simulink model "ModeS_testbench_org"  (Simulink 10.0)
settings: Solver=VariableStepDiscrete  StartTime=0.0  StopTime=1e6  RelTol=1e-3
PreLoadFcn:
  | load data_Yb;
  | 
  | DataIn = Yb_with_time(:,2);
  | 
  | wl=16;
undefined symbols (not defined in the file): dfilt
libraries: simulink x27, dspobslib x2, dspsnks4 x2, hdlsllib x1, dspindex x1, dspsrcs4 x1
settings Model: Creator=mdonovan  LastModifiedBy=annonymous
settings DataIOCC: LimitDataPoints=on  SignalLoggingSaveFormat=ModelDataLogs  SaveOutput=off  SignalLogging=off  SaveTime=off
settings OptimizationCC: BlockReduction=off  BooleanDataType=off  ConditionallyExecuteInputs=off  DefaultParameterBehavior=Inlined  ExpressionDepthLimit=2147483647  LocalBlockOutputs=off
settings DebuggingCC: AlgebraicLoopMsg=error  SolverPrmCheckMsg=warning  SingleTaskRateTransMsg=error  FcnCallInpInsideContextMsg=warning  AllowSymbolicDim=off  StateNameClashWarn=warning
settings HardwareCC: ProdHWDeviceType=ASIC/FPGA->ASIC/FPGA  TargetBitPerLong=64  TargetBitPerPointer=64  TargetBitPerSizeT=64  TargetBitPerPtrDiffT=64  TargetLongLongMode=on  TargetIntDivRoundTo=Zero  TargetEndianess=LittleEndian  TargetWordSize=64  TargetHWDeviceType=MATLAB Host  ProdEqTarget=off
settings GRTTargetCC: GeneratePreprocessorConditionals=Disable all
settings ConfigComp: CovExternalEMLEnable=off

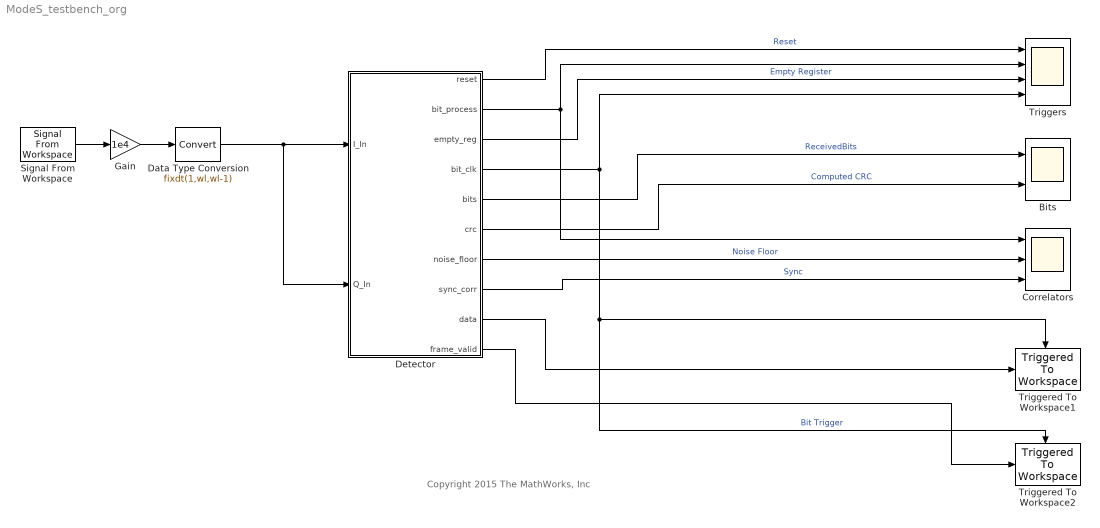
== system ModeS_testbench_org ==
  note: Copyright 2015 The MathWorks, Inc
  Bits : Scope  NumInputPorts=2
  Correlators : Scope  NumInputPorts=3
  Data Type Conversion : DataTypeConversion  OutDataTypeStr=fixdt(1,wl,wl-1)  LockScale=on
  Detector : Subsystem  TreatAsAtomicUnit=on
  Gain : Gain  Gain=1e4
  Signal From Workspace : dspsrcs4/Signal From Workspace  X=DataIn  Ts=1  nsamps=1  OutputAfterFinalValue=Setting to zero  ignoreOrWarnInputAndFrameLengths=off  OutputFrames=on
  Triggered To Workspace1 : dspsnks4/Triggered To Workspace  TriggerType=Rising edge  VariableName=data_out  Buffer=1000  Save2DMode=2-D array (concatenate along first dimension)
      settings: SourceProductName=DSP System Toolbox  SourceProductBaseCode=DS  FixptAsFi=off
  Triggered To Workspace2 : dspsnks4/Triggered To Workspace  TriggerType=Rising edge  VariableName=frame_valid  Buffer=1000  Save2DMode=2-D array (concatenate along first dimension)
      settings: SourceProductName=DSP System Toolbox  SourceProductBaseCode=DS  FixptAsFi=off
  Triggers : Scope  NumInputPorts=4
  wires:
  Signal From Workspace/1 -> Gain/1
  Data Type Conversion/1 -> Detector/1(I_In), Detector/2(Q_In)
  Gain/1 -> Data Type Conversion/1
  Detector/5(bits) -> Bits/1  "ReceivedBits"
  Detector/4(bit_clk) -> Triggered To Workspace2/Trigger, Triggered To Workspace1/Trigger, Triggers/4  "Bit Trigger"
  Detector/10(frame_valid) -> Triggered To Workspace2/1
  Detector/9(data) -> Triggered To Workspace1/1
  Detector/7(noise_floor) -> Correlators/2  "Noise Floor"
  Detector/6(crc) -> Bits/2  "Computed CRC"
  Detector/1(reset) -> Triggers/1  "Reset"
  Detector/2(bit_process) -> Triggers/2, Correlators/1
  Detector/3(empty_reg) -> Triggers/3  "Empty Register"
  Detector/8(sync_corr) -> Correlators/3  "Sync"

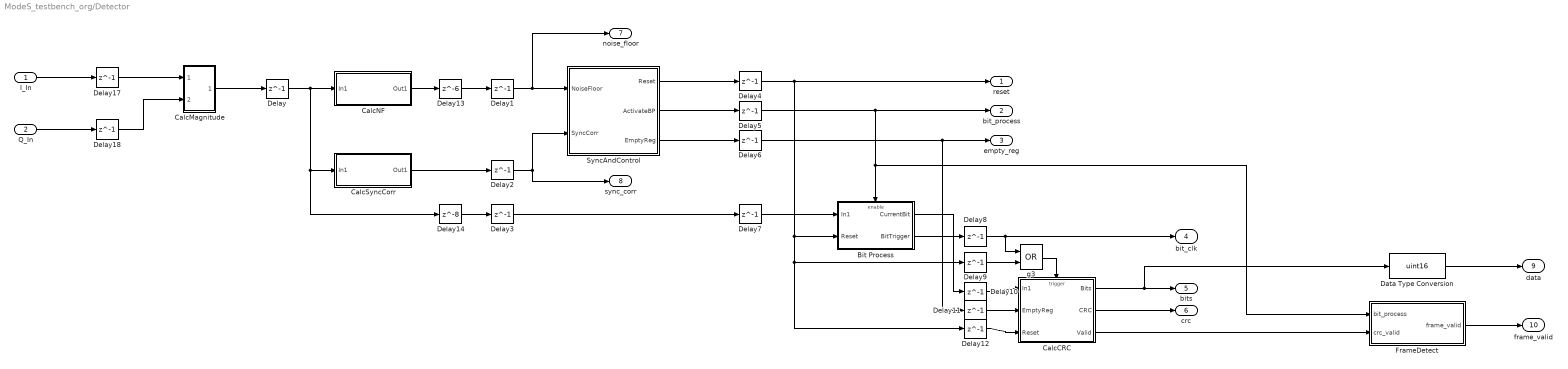
== system ModeS_testbench_org/Detector ==
  I_In : Inport
  Q_In : Inport  Port=2
  Bit Process : Subsystem  TreatAsAtomicUnit=on
  CalcCRC : Subsystem
  CalcMagnitude : Subsystem
  CalcNF : Subsystem
  CalcSyncCorr : Subsystem
  Data Type Conversion : DataTypeConversion  OutDataTypeStr=uint16
  Delay{,1..12,17..18} (15 alike) : Delay  DelayLength=1  InitialCondition=0  InputProcessing=Columns as channels (frame based)
  Delay13 : Delay  DelayLength=6  InitialCondition=0  InputProcessing=Columns as channels (frame based)
  Delay14 : Delay  DelayLength=8  InitialCondition=0  InputProcessing=Columns as channels (frame based)
  FrameDetect : Subsystem
  SyncAndControl : Stateflow chart  TreatAsAtomicUnit=on
  g3 : Logic  Operator=OR  AllPortsSameDT=off  OutDataTypeStr=boolean
  reset : Outport  VectorParamsAs1DForOutWhenUnconnected=off
  bit_process : Outport  Port=2  VectorParamsAs1DForOutWhenUnconnected=off
  empty_reg : Outport  Port=3  VectorParamsAs1DForOutWhenUnconnected=off
  bit_clk : Outport  Port=4  VectorParamsAs1DForOutWhenUnconnected=off
  bits : Outport  Port=5  VectorParamsAs1DForOutWhenUnconnected=off
  crc : Outport  Port=6  VectorParamsAs1DForOutWhenUnconnected=off
  noise_floor : Outport  Port=7  VectorParamsAs1DForOutWhenUnconnected=off
  sync_corr : Outport  Port=8  VectorParamsAs1DForOutWhenUnconnected=off
  data : Outport  Port=9  VectorParamsAs1DForOutWhenUnconnected=off
  frame_valid : Outport  Port=10  VectorParamsAs1DForOutWhenUnconnected=off
  wires:
  SyncAndControl/1(Reset) -> Delay4/1
  Bit Process/1(CurrentBit) -> Delay10/1
  SyncAndControl/3(EmptyReg) -> Delay6/1
  SyncAndControl/2(ActivateBP) -> Delay5/1
  Bit Process/2(BitTrigger) -> Delay8/1
  g3/1 -> CalcCRC/Trigger
  CalcNF/1(Out1) -> Delay13/1
  CalcSyncCorr/1(Out1) -> Delay2/1
  CalcCRC/1(Bits) -> Data Type Conversion/1, bits/1
  CalcCRC/2(CRC) -> crc/1
  Delay1/1 -> SyncAndControl/1(NoiseFloor), noise_floor/1
  Delay2/1 -> SyncAndControl/2(SyncCorr), sync_corr/1
  Delay3/1 -> Delay7/1
  Delay4/1 -> reset/1, Delay9/1, Delay12/1, Bit Process/2(Reset)
  Delay5/1 -> FrameDetect/1(bit_process), Bit Process/Enable, bit_process/1
  Delay6/1 -> empty_reg/1, Delay11/1
  Delay7/1 -> Bit Process/1(In1)
  Delay10/1 -> CalcCRC/1(In1)
  Delay11/1 -> CalcCRC/2(EmptyReg)
  Delay13/1 -> Delay1/1
  I_In/1 -> Delay17/1
  Q_In/1 -> Delay18/1
  Delay17/1 -> CalcMagnitude/1(In1)
  Delay18/1 -> CalcMagnitude/2(In2)
  CalcMagnitude/1(Out1) -> Delay/1
  Delay8/1 -> g3/1, bit_clk/1
  Delay12/1 -> CalcCRC/3(Reset)
  Delay9/1 -> g3/2
  CalcCRC/3(Valid) -> FrameDetect/2(crc_valid)
  FrameDetect/1(frame_valid) -> frame_valid/1
  Data Type Conversion/1 -> data/1
  Delay/1 -> CalcNF/1(In1), Delay14/1, CalcSyncCorr/1(In1)
  Delay14/1 -> Delay3/1

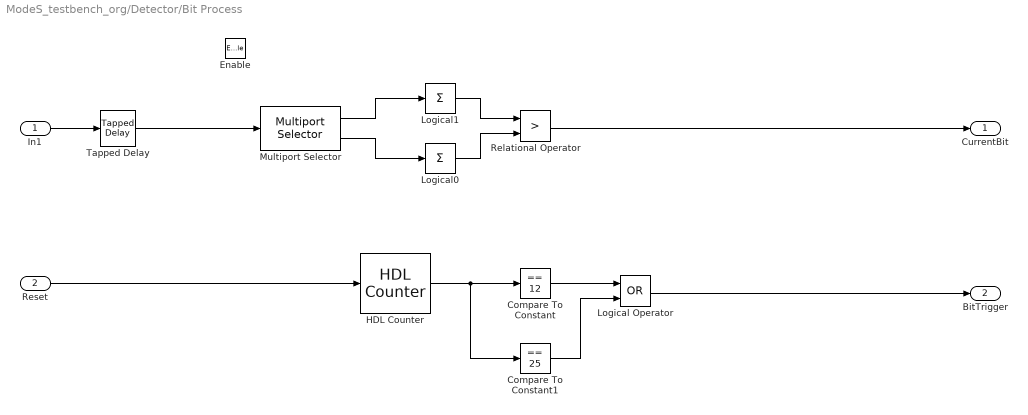
== system ModeS_testbench_org/Detector/Bit Process ==
  In1 : Inport
  Reset : Inport  Port=2
  Enable : EnablePort
  Compare To Constant : simulink/Logic and Bit Operations/Compare To Constant  relop===  const=12  OutDataTypeStr=boolean
  Compare To Constant1 : simulink/Logic and Bit Operations/Compare To Constant  relop===  const=25  OutDataTypeStr=boolean
  HDL Counter : hdlsllib/HDL Operations/HDL Counter  CountType=Count limited  CountInit=1  CountStep=1  CountMax=25  CountFromType=Initial value  CountFrom=1  CountResetPort=on  CountLoadPort=off  CountEnbPort=off  CountDirPort=off  CountDataType=Unsigned  CountWordLen=8  CountFracLen=0  CountSampTime=1
      settings: SourceProductName=HDL Coder  SourceProductBaseCode=HD
  Logical Operator : Logic  Operator=OR  AllPortsSameDT=off  OutDataTypeStr=boolean
  Logical0 : Sum  Inputs=+  AccumDataTypeStr=fixdt(1,wl,wl-3)  OutDataTypeStr=Inherit: Same as accumulator
  Logical1 : Sum  Inputs=+  AccumDataTypeStr=fixdt(1,wl,wl-3)  OutDataTypeStr=Inherit: Same as accumulator
  Multiport Selector : dspindex/Multiport Selector  rowsOrCols=Rows  idxCellArray={ 1:6,7:12}  idxErrMode=Clip Index
  Relational Operator : RelationalOperator  Operator=>  OutDataTypeStr=boolean  RndMeth=Nearest
  Tapped Delay : simulink/Discrete/Tapped Delay  vinit=0.0  samptime=1  NumDelays=12  DelayOrder=Oldest  includeCurrent=on
  CurrentBit : Outport  InitialOutput=0  VectorParamsAs1DForOutWhenUnconnected=off
  BitTrigger : Outport  Port=2  InitialOutput=0  VectorParamsAs1DForOutWhenUnconnected=off
  wires:
  Tapped Delay/1 -> Multiport Selector/1
  Multiport Selector/1 -> Logical1/1
  Multiport Selector/2 -> Logical0/1
  Logical1/1 -> Relational Operator/1
  Logical0/1 -> Relational Operator/2
  In1/1 -> Tapped Delay/1
  Relational Operator/1 -> CurrentBit/1
  Reset/1 -> HDL Counter/1
  HDL Counter/1 -> Compare To Constant/1, Compare To Constant1/1
  Compare To Constant/1 -> Logical Operator/1
  Compare To Constant1/1 -> Logical Operator/2
  Logical Operator/1 -> BitTrigger/1

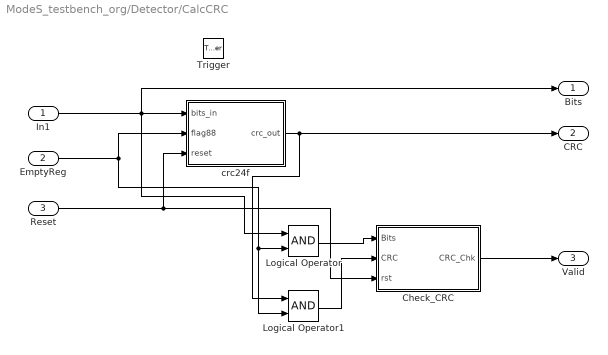
== system ModeS_testbench_org/Detector/CalcCRC ==
  In1 : Inport
  EmptyReg : Inport  Port=2
  Reset : Inport  Port=3
  Trigger : TriggerPort  VariantControl=Variant
  Check_CRC : Subsystem  TreatAsAtomicUnit=on
  Logical Operator : Logic  AllPortsSameDT=off  OutDataTypeStr=boolean
  Logical Operator1 : Logic  AllPortsSameDT=off  OutDataTypeStr=boolean
  crc24f : Subsystem
  Bits : Outport  InitialOutput=0  VectorParamsAs1DForOutWhenUnconnected=off
  CRC : Outport  Port=2  InitialOutput=0  VectorParamsAs1DForOutWhenUnconnected=off
  Valid : Outport  Port=3  InitialOutput=0  VectorParamsAs1DForOutWhenUnconnected=off
  wires:
  In1/1 -> Bits/1, Logical Operator/1, crc24f/1(bits_in)
  EmptyReg/1 -> crc24f/2(flag88), Logical Operator1/2, Logical Operator/2
  crc24f/1(crc_out) -> Logical Operator1/1, CRC/1
  Reset/1 -> Check_CRC/3(rst), crc24f/3(reset)
  Logical Operator/1 -> Check_CRC/1(Bits)
  Logical Operator1/1 -> Check_CRC/2(CRC)
  Check_CRC/1(CRC_Chk) -> Valid/1

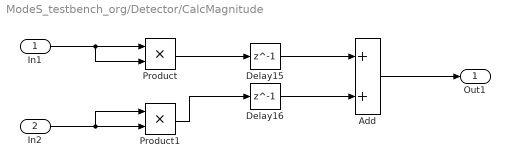
== system ModeS_testbench_org/Detector/CalcMagnitude ==
  In1 : Inport
  In2 : Inport  Port=2
  Add : Sum  OutDataTypeStr=fixdt(1,wl,wl-1)
  Delay15 : Delay  DelayLength=1  InitialCondition=0  InputProcessing=Columns as channels (frame based)
  Delay16 : Delay  DelayLength=1  InitialCondition=0  InputProcessing=Columns as channels (frame based)
  Product : Product  OutDataTypeStr=fixdt(1,wl,wl-1)
  Product1 : Product  OutDataTypeStr=fixdt(1,wl,wl-1)
  Out1 : Outport  VectorParamsAs1DForOutWhenUnconnected=off
  wires:
  Product/1 -> Delay15/1
  Product1/1 -> Delay16/1
  In1/1 -> Product/2, Product/1
  In2/1 -> Product1/1, Product1/2
  Delay15/1 -> Add/1
  Add/1 -> Out1/1
  Delay16/1 -> Add/2

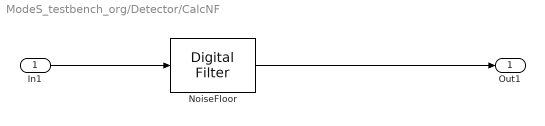
== system ModeS_testbench_org/Detector/CalcNF ==
  In1 : Inport
  NoiseFloor : dspobslib/Digital Filter  TypePopup=FIR (all zeros)  IIRFiltStruct=Direct form II transposed  AllPoleFiltStruct=Direct form  FIRFiltStruct=Direct form transposed  CoeffSource=Specify via dialog  NumCoeffs=(ones(64,1)/64)  DenCoeffs=[1 0.1]  BiQuadCoeffs=[1 0.3 0.4 1 0.1 0.2]  LatticeCoeffs=[0.2 0.4]  denIgnore=on  FiltPerSampPopup=One filter per frame  IC=0  ICnum=0  ICden=0  firstCoeffMode=Binary point scaling  firstCoeffWordLength=wl  firstCoeffFracLength=wl+4  outputMode=Binary point scaling  outputWordLength=wl  outputFracLength=wl  accumMode=Binary point scaling  accumWordLength=wl*2  accumFracLength=wl*2  prodOutputMode=Binary point scaling  prodOutputWordLength=wl*2  prodOutputFracLength=wl*2+5  roundingMode=Floor  overflowMode=off  ScaleValues=1  scaleValueFracLength=14  stageInFracLength=15  stageOutFracLength=15  FilterSource=Specify via dialog  dfiltObjectName=dfilt.dffir([1 2 1])  InputProcessing=Columns as channels (frame based)
      settings: SourceProductName=DSP System Toolbox  SourceProductBaseCode=DS
  Out1 : Outport  VectorParamsAs1DForOutWhenUnconnected=off
  wires:
  In1/1 -> NoiseFloor/1
  NoiseFloor/1 -> Out1/1

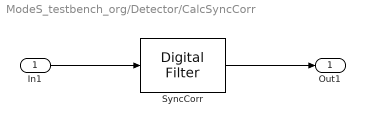
== system ModeS_testbench_org/Detector/CalcSyncCorr ==
  In1 : Inport
  SyncCorr : dspobslib/Digital Filter  TypePopup=FIR (all zeros)  IIRFiltStruct=Direct form II transposed  AllPoleFiltStruct=Direct form  FIRFiltStruct=Direct form  CoeffSource=Specify via dialog  NumCoeffs=|  DenCoeffs=[1 0.1]  BiQuadCoeffs=[1 0.3 0.4 1 0.1 0.2]  LatticeCoeffs=[0.2 0.4]  denIgnore=on  FiltPerSampPopup=One filter per frame  IC=0  ICnum=0  ICden=0  firstCoeffMode=Binary point scaling  firstCoeffWordLength=wl  firstCoeffFracLength=wl-2  outputMode=Binary point scaling  outputWordLength=wl  outputFracLength=wl-5  accumMode=Binary point scaling  accumWordLength=wl*2  accumFracLength=wl*2-5  prodOutputMode=Binary point scaling  prodOutputWordLength=wl*2  prodOutputFracLength=wl*2-1  roundingMode=Floor  overflowMode=off  ScaleValues=1  scaleValueFracLength=14  stageInFracLength=15  stageOutFracLength=15  FilterSource=Specify via dialog  dfiltObjectName=dfilt.dffir([1 2 1])  InputProcessing=Columns as channels (frame based)
      | flipud([ones(6,1);-1*ones(6,1);ones(6,1);-1*ones(7,1);
      | -1*ones(6,1);-1*ones(6,1);-1*ones(6,1);ones(7,1);-1*ones(6,1);ones(6,1);-1*ones(6,1);-1*ones(7,1)])
      settings: SourceProductName=DSP System Toolbox  SourceProductBaseCode=DS
  Out1 : Outport  VectorParamsAs1DForOutWhenUnconnected=off
  wires:
  In1/1 -> SyncCorr/1
  SyncCorr/1 -> Out1/1

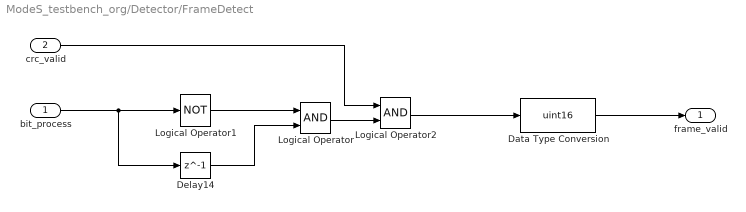
== system ModeS_testbench_org/Detector/FrameDetect ==
  bit_process : Inport
  crc_valid : Inport  Port=2
  Data Type Conversion : DataTypeConversion  OutDataTypeStr=uint16
  Delay14 : Delay  DelayLength=1  InitialCondition=0  InputProcessing=Columns as channels (frame based)
  Logical Operator : Logic  AllPortsSameDT=off  OutDataTypeStr=boolean
  Logical Operator1 : Logic  Operator=NOT  AllPortsSameDT=off  OutDataTypeStr=boolean
  Logical Operator2 : Logic  AllPortsSameDT=off  OutDataTypeStr=boolean
  frame_valid : Outport  VectorParamsAs1DForOutWhenUnconnected=off
  wires:
  crc_valid/1 -> Logical Operator2/1
  Logical Operator/1 -> Logical Operator2/2
  Logical Operator1/1 -> Logical Operator/1
  Delay14/1 -> Logical Operator/2
  bit_process/1 -> Delay14/1, Logical Operator1/1
  Logical Operator2/1 -> Data Type Conversion/1
  Data Type Conversion/1 -> frame_valid/1

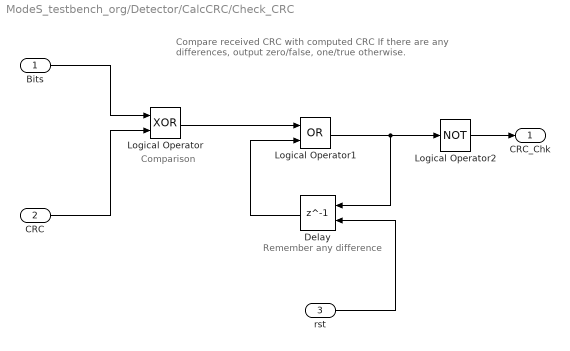
== system ModeS_testbench_org/Detector/CalcCRC/Check_CRC ==
  note: Compare received CRC with computed CRC
      | If there are any differences, output zero/false, one/true otherwise.
  note: Comparison
  note: Remember any difference
  Bits : Inport
  CRC : Inport  Port=2
  rst : Inport  Port=3
  Delay : Delay  DelayLength=1  ExternalReset=Level
      settings: InputPortMap=u0,r5
  Logical Operator : Logic  Operator=XOR  AllPortsSameDT=off  OutDataTypeStr=boolean
  Logical Operator1 : Logic  Operator=OR  AllPortsSameDT=off  OutDataTypeStr=boolean
  Logical Operator2 : Logic  Operator=NOT  AllPortsSameDT=off  OutDataTypeStr=boolean
  CRC_Chk : Outport  InitialOutput=0  VectorParamsAs1DForOutWhenUnconnected=off
  wires:
  Bits/1 -> Logical Operator/1
  CRC/1 -> Logical Operator/2
  Logical Operator/1 -> Logical Operator1/1
  Delay/1 -> Logical Operator1/2
  Logical Operator1/1 -> Delay/1, Logical Operator2/1
  Logical Operator2/1 -> CRC_Chk/1
  rst/1 -> Delay/2

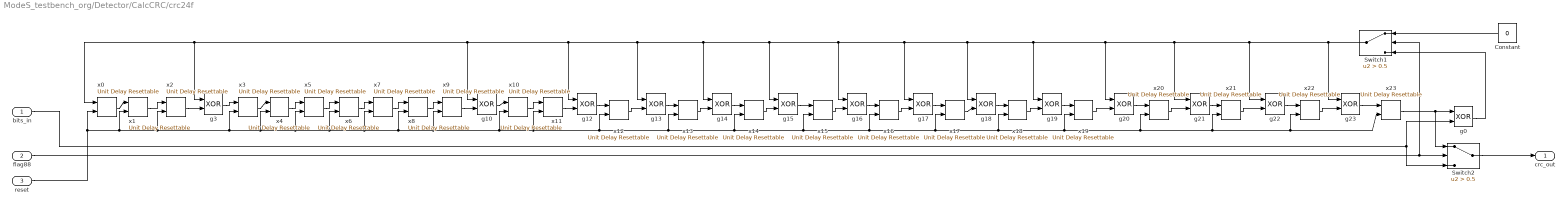
== system ModeS_testbench_org/Detector/CalcCRC/crc24f ==
  bits_in : Inport
  flag88 : Inport  Port=2
  reset : Inport  Port=3
  Constant : Constant  Value=0  OutDataTypeStr=boolean  SampleTime=-1
  Switch1 : Switch  Criteria=u2 > Threshold  Threshold=0.5
  Switch2 : Switch  Criteria=u2 > Threshold  Threshold=0.5
  g{0,3,10,12..23} (15 alike) : Logic  Operator=XOR  AllPortsSameDT=off  OutDataTypeStr=boolean
  x{0..23} (24 alike) : simulink/Additional Math & Discrete/Additional Discrete/Unit Delay Resettable  vinit=0.0  tsamp=-1
      settings: SourceProductName=Simulink  SourceProductBaseCode=SL
  crc_out : Outport  VectorParamsAs1DForOutWhenUnconnected=off
  wires:
  x0/1 -> x1/1
  x1/1 -> x2/1
  x3/1 -> x4/1
  x4/1 -> x5/1
  x5/1 -> x6/1
  x6/1 -> x7/1
  x7/1 -> x8/1
  x8/1 -> x9/1
  x10/1 -> x11/1
  g3/1 -> x3/1
  x2/1 -> g3/2
  g10/1 -> x10/1
  x9/1 -> g10/2
  x11/1 -> g12/2
  g12/1 -> x12/1
  x12/1 -> g13/2
  g13/1 -> x13/1
  x13/1 -> g14/2
  g14/1 -> x14/1
  x14/1 -> g15/2
  g15/1 -> x15/1
  x15/1 -> g16/2
  g16/1 -> x16/1
  x16/1 -> g17/2
  g17/1 -> x17/1
  x17/1 -> g18/2
  g18/1 -> x18/1
  x18/1 -> g19/2
  g19/1 -> x19/1
  x19/1 -> g20/2
  g20/1 -> x20/1
  x20/1 -> g21/2
  g21/1 -> x21/1
  x21/1 -> g22/2
  g22/1 -> x22/1
  x22/1 -> g23/2
  g23/1 -> x23/1
  bits_in/1 -> g0/2, Switch2/3
  Switch2/1 -> crc_out/1
  flag88/1 -> Switch2/2, Switch1/2
  x23/1 -> g0/1, Switch2/1
  Switch1/1 -> g10/1, g3/1, x0/1, g12/1, g13/1, g14/1, g15/1, g16/1, g17/1, g18/1, g19/1, g20/1, g21/1, g22/1, g23/1
  reset/1 -> x0/2, x1/2, x2/2, x3/2, x4/2, x5/2, x6/2, x7/2, x8/2, x9/2, x10/2, x11/2, x12/2, x13/2, x14/2, x15/2, x16/2, x17/2, x18/2, x19/2, x20/2, x21/2, x22/2, x23/2
  Constant/1 -> Switch1/1
  g0/1 -> Switch1/3

== stateflow chart Detector/SyncAndControl ==
  settings: executeAtInitialization=1
  state SyncSearch
  state WaitForT0
    entry: T0Delay++;
  state BitProcess
    entry: SamplesIn++;
    Reset = 0;
  state ClearBP
    entry: SamplesIn++;
  state EmptyReg
    entry: CRCClocks++;
  (default) -> SyncSearch
  ClearBP -> SyncSearch [order 1] : [SamplesIn>100]
  SyncSearch -> WaitForT0 : [SyncCorr > 40*NoiseFloor]
      | {ActivateBP = 1;
      | maxSync = SyncCorr;
      | SamplesIn = 0;
      | T0Delay = 0;
      | Reset = 1;}
  WaitForT0 -> WaitForT0 [order 3]
  BitProcess -> WaitForT0 [order 2] : [SyncCorr > maxSync && SamplesIn < 50]
      | {Reset = 1;
      | SamplesIn = 0;
      | maxSync = SyncCorr;
      | T0Delay = 0;}
  WaitForT0 -> WaitForT0 [order 2] : [SyncCorr > maxSync]
      | {T0Delay = 0;
      | maxSync = SyncCorr;}
  WaitForT0 -> BitProcess [order 1] : [T0Delay>25]
  BitProcess -> BitProcess [order 3]
  ClearBP -> ClearBP [order 2]
  BitProcess -> EmptyReg [order 1] : [SamplesIn>=12.5*88]
      | {EmptyReg = 1;
      | CRCClocks = 0;}
  EmptyReg -> ClearBP [order 1] : [CRCClocks>=24*12.5]
      | {maxSync = 0;
      | ActivateBP = 0;
      | Reset = 0;
      | SamplesIn = 0;
      | EmptyReg = 0;}
  EmptyReg -> EmptyReg [order 2]
  data: NoiseFloor input double; SyncCorr input double; Reset output boolean =0; ActivateBP output boolean =0; EmptyReg output boolean =0; SamplesIn local uint16 =0; maxSync local fixdt(1,14,9) =0; CRCClocks local uint16 =0; T0Delay local uint8 =0
